simulink model "auto_pilot_upl"  (R2022b)
settings: Solver=FixedStepAuto  StartTime=0.0  StopTime=Inf  FixedStep=0.001  RelTol=1e-3  EnableMultiTasking=on
InitFcn:
  | clear mex
model workspace (MAT data in the model file):
  worldsim_instance : object (value not decoded)
values from neighbouring files (symbols this model uses):
  ACC_Adaptive_D = 0    [AutoPilot_parameters.m]    (also in ap_ini_param.mat; ap_initialModel.sldd = 0.0)
  ACC_Adaptive_I = 0    [AutoPilot_parameters.m]    (also in ap_ini_param.mat; ap_initialModel.sldd = 0.0)
  ACC_Adaptive_P = [5 7.5]    [AutoPilot_parameters.m]    (also in ap_ini_param.mat; ap_initialModel.sldd = 5.0 7.5)
  ACC_Classic_I = 5    [AutoPilot_parameters.m]    (also in ap_ini_param.mat; ap_initialModel.sldd = 5.0)
  ACC_Classic_P = 15    [AutoPilot_parameters.m]    (also in ap_ini_param.mat; ap_initialModel.sldd = 15.0)
  ACC_MaxBrake = 50    [AutoPilot_parameters.m]    (also in ap_ini_param.mat; ap_initialModel.sldd = 50.0)
  ACC_MaxThrottle = 130    [AutoPilot_parameters.m]    (also in ap_ini_param.mat = 80; ap_initialModel.sldd = 130.0)
  ACC_Module_Activity_Flag = 1    [AutoPilot_parameters.m]    (also in ap_ini_param.mat; ap_initialModel.sldd = 1.0)
  ACC_Ready_Speed = 30    [AutoPilot_parameters.m]    (also in ap_ini_param.mat; ap_initialModel.sldd = 30.0)
  ACC_SensorMaxDistance = 250    [AutoPilot_parameters.m]    (also in ap_ini_param.mat = 120; ap_initialModel.sldd = 250.0)
  ACC_Speed_Distance_control = 3    [AutoPilot_parameters.m]    (also in ap_ini_param.mat; ap_initialModel.sldd = 3.0)
  ACC_Speed_Distance_Gain = [0.1 0.15 0.2 0.25]    [AutoPilot_parameters.m]    (also in ap_ini_param.mat; ap_initialModel.sldd = 0.1 0.15 0.2 0.25)
  ADAS_Control_Mode = 1    [AutoPilot_parameters.m]    (also in ap_ini_param.mat; ap_initialModel.sldd = 1.0)
  AEB_Alarm_Freq = 5    [AutoPilot_parameters.m]    (also in ap_ini_param.mat; ap_initialModel.sldd = 5.0)
  AEB_Distance_To_Collision_Brake = 5    [AutoPilot_parameters.m]    (also in ap_ini_param.mat; ap_initialModel.sldd = 5.0)
  AEB_Freq_Hz = Sensor_Freq_worldsim/2    (= 25)    [AutoPilot_parameters.m]    (also in ap_ini_param.mat; ap_initialModel.sldd = 25.0)
  AEB_Gain = [1 1]    [AutoPilot_parameters.m]    (also in ap_ini_param.mat; ap_initialModel.sldd = 1.0 1.0)
  AEB_Gain_set = 60    [AutoPilot_parameters.m]    (also in ap_ini_param.mat; ap_initialModel.sldd = 60.0)
  AEB_Gain_set_mult = 0.03    [AutoPilot_parameters.m]    (also in ap_ini_param.mat; ap_initialModel.sldd)
  AEB_Max_Decel = [8 15]    [AutoPilot_parameters.m]    (also in ap_ini_param.mat; ap_initialModel.sldd = 8.0 15.0)
  AEB_Max_Speed = 150    [AutoPilot_parameters.m]    (also in ap_ini_param.mat = 100; ap_initialModel.sldd = 150.0)
  AEB_Min_Distance_at_Stop = 1    [AutoPilot_parameters.m]    (also in ap_ini_param.mat; ap_initialModel.sldd = 1.0)
  AEB_Module_Activity_Flag = 1    [AutoPilot_parameters.m]    (also in ap_ini_param.mat; ap_initialModel.sldd = 1.0)
  AEB_Pedestrian_type = 68    [AutoPilot_parameters.m]    (also in ap_ini_param.mat; ap_initialModel.sldd = 68.0)
  AEB_Steer_Max = 180    [AutoPilot_parameters.m]    (also in ap_ini_param.mat; ap_initialModel.sldd = 180.0)
  AP_Activity_Flag = 1    [AutoPilot_parameters.m]    (also in ap_ini_param.mat; ap_initialModel.sldd = 1.0)
  AP_D = [0.3 0.3]    [AutoPilot_parameters.m]    (also in ap_ini_param.mat; ap_initialModel.sldd = 0.3 0.3)
  AP_Dyn_Rate_Limiter_Gain = 0.1    [AutoPilot_parameters.m]    (also in ap_ini_param.mat; ap_initialModel.sldd)
  AP_Dyn_Rate_Limiter_Power = 10    [AutoPilot_parameters.m]    (also in ap_ini_param.mat; ap_initialModel.sldd = 10.0)
  AP_Error_Max = 3    [AutoPilot_parameters.m]    (also in ap_ini_param.mat; ap_initialModel.sldd = 3.0)
  AP_Freq_Hz = Sensor_Freq_worldsim    (= 50)    [AutoPilot_parameters.m]    (also in ap_ini_param.mat; ap_initialModel.sldd = 50.0)
  AP_I = [0.05 0.05]    [AutoPilot_parameters.m]    (also in ap_ini_param.mat; ap_initialModel.sldd = 0.05 0.05)
  AP_Max_Error_dydt_Disable = 0.5    [AutoPilot_parameters.m]    (also in ap_ini_param.mat; ap_initialModel.sldd)
  AP_On_Request_Time = 0.01    [AutoPilot_parameters.m]    (also in ap_ini_param.mat; ap_initialModel.sldd)
  AP_P = [0.2 0.2]    [AutoPilot_parameters.m]    (also in ap_ini_param.mat; ap_initialModel.sldd = 0.2 0.2)
  AP_Steer_Error_Max = 0.7    [AutoPilot_parameters.m]    (also in ap_ini_param.mat; ap_initialModel.sldd)
  AP_Steer_Rate_Max_radps = 1    [AutoPilot_parameters.m]    (also in ap_ini_param.mat; ap_initialModel.sldd = 1.0)
  AP_Transition_Rate = 0.5    [AutoPilot_parameters.m]    (also in ap_ini_param.mat; ap_initialModel.sldd)
  butter_a = [1 -1.9911142922 0.991153595869]    [ap_ini_param.mat]    (also in ap_initialModel.sldd = 1.0 -1.9911142922016536 0.99115359586893548)
  butter_b = [9.82591682048e-06 1.9651833641e-05 9.82591682048e-06]    [ap_ini_param.mat]    (also in ap_initialModel.sldd = 9.825916820482009E-6 1.9651833640964018E-5 9.825916820482009)
  Lane_Width = 3.7    [AutoPilot_parameters.m]    (also in ap_ini_param.mat; ap_initialModel.sldd)
  No_Target_Display_Value = 0    [AutoPilot_parameters.m]    (also in ap_ini_param.mat; ap_initialModel.sldd = 0.0)
  radar_source = 2    [AutoPilot_parameters.m]    (also in ap_ini_param.mat; ap_initialModel.sldd = 2.0)
  Sensor_Freq_worldsim = 50    [AutoPilot_parameters.m]    (also in ap_ini_param.mat; ap_initialModel.sldd = 50.0; launcher.m)
  stop_number_collisions = 10.0    [ap_initialModel.sldd]    (also in launcher.m = 10)
  stop_speed = 0.001    [ap_initialModel.sldd]    (also in launcher.m)
  stop_time = 12.0    [ap_initialModel.sldd]    (also in launcher.m = 12)
  vehicle_width = 2.2    [AutoPilot_parameters.m]    (also in ap_ini_param.mat = 1.86; ap_initialModel.sldd)
undefined symbols (not defined in the file or in its folder): light_brake_center, light_brake_left, light_brake_right
libraries: simulink x91, simwbSfunlib x49, viworldsim_lib x6, slpidlib x4
(part 4 of 4)

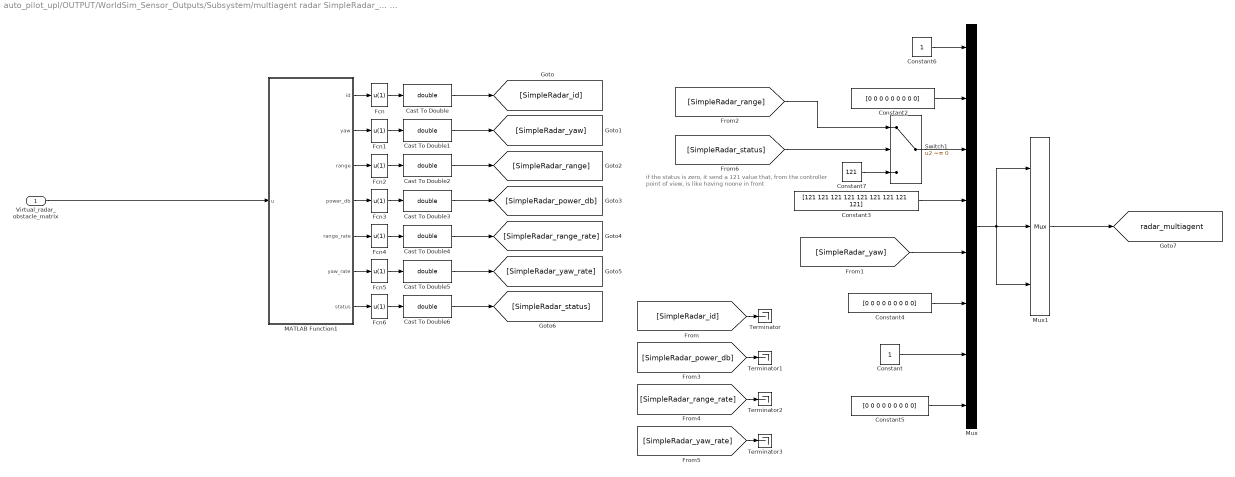
== system auto_pilot_upl/OUTPUT/WorldSim_Sensor_Outputs/Subsystem/multiagent radar SimpleRadar_... are single double representing id, yaw, range, power_db, range_rate, yaw_rate, status ==
  note: if the status is zero, it send a 121 value that,
      | from the controller point of view, is like having noone in front
  Virtual_radar_obstacle_matrix : Inport
  Cast To Double{,1..6} (7 alike) : DataTypeConversion  OutDataTypeStr=double  SaturateOnIntegerOverflow=off  RndMeth=Floor
  Constant : Constant
  Constant2 : Constant  Value=[0 0 0 0 0 0 0 0 0]
  Constant3 : Constant  Value=[121 121 121 121 121 121 121 121 121]
  Constant4 : Constant  Value=[0 0 0 0 0 0 0 0 0]
  Constant5 : Constant  Value=[0 0 0 0 0 0 0 0 0]
  Constant6 : Constant
  Constant7 : Constant  Value=121
  Fcn{,1..6} (7 alike) : Fcn  Expr=u(1)
  MATLAB Function1 : MATLAB Function  TreatAsAtomicUnit=on
  Mux : Mux  Inputs=8
  Mux1 : Mux  Inputs=3
  Switch1 : Switch  Criteria=u2 ~= 0  SaturateOnIntegerOverflow=off  InputSameDT=off
  Terminator{,1..3} (4 alike) : Terminator
  tag scope: radar_multiagent=global
  wires:
  Virtual_radar_obstacle_matrix/1 -> MATLAB Function1/1(u)
  MATLAB Function1/6(yaw_rate) -> Fcn5/1
  Cast To Double3/1 -> [SimpleRadar_power_db]
  Cast To Double5/1 -> [SimpleRadar_yaw_rate]
  MATLAB Function1/1(id) -> Fcn/1
  Fcn4/1 -> Cast To Double4/1
  Cast To Double2/1 -> [SimpleRadar_range]
  Fcn5/1 -> Cast To Double5/1
  MATLAB Function1/2(yaw) -> Fcn1/1
  Cast To Double/1 -> [SimpleRadar_id]
  MATLAB Function1/7(status) -> Fcn6/1
  Fcn1/1 -> Cast To Double1/1
  Fcn6/1 -> Cast To Double6/1
  Fcn/1 -> Cast To Double/1
  Cast To Double4/1 -> [SimpleRadar_range_rate]
  MATLAB Function1/5(range_rate) -> Fcn4/1
  Cast To Double1/1 -> [SimpleRadar_yaw]
  MATLAB Function1/4(power_db) -> Fcn3/1
  Fcn2/1 -> Cast To Double2/1
  Fcn3/1 -> Cast To Double3/1
  MATLAB Function1/3(range) -> Fcn2/1
  Cast To Double6/1 -> [SimpleRadar_status]
  Switch1/1 -> Mux/3
  [SimpleRadar_yaw] -> Mux/5
  [SimpleRadar_status] -> Switch1/2
  Constant3/1 -> Mux/4
  Mux/1 -> Mux1/3, Mux1/1, Mux1/2
  Constant5/1 -> Mux/8
  Constant6/1 -> Mux/1
  Constant/1 -> Mux/7
  Constant4/1 -> Mux/6
  [SimpleRadar_yaw_rate] -> Terminator3/1
  Constant7/1 -> Switch1/3
  Constant2/1 -> Mux/2
  [SimpleRadar_range_rate] -> Terminator2/1
  [SimpleRadar_range] -> Switch1/1
  Mux1/1 -> [radar_multiagent]
  [SimpleRadar_id] -> Terminator/1
  [SimpleRadar_power_db] -> Terminator1/1

== system auto_pilot_upl/OUTPUT/WorldSim_Sensor_Outputs/Subsystem/obstacle detection  ==
  Virtual_camera_obstacle_matrix : Inport
  From1 : From  Commented=on  GotoTag=Obstacles_id
  Gain : Gain  Gain=0.5
  MATLAB Function : MATLAB Function  TreatAsAtomicUnit=on
  MATLAB Function2 : MATLAB Function  TreatAsAtomicUnit=on
  Mux2 : Mux
  Mux3 : Mux  Inputs=3
  Sum : Sum  Inputs=+-
  Terminator{,4..8} (6 alike) : Terminator
  tag scope: Obstacles_nearest_point_x=global, Obstacles_nearest_point_y=global, Obstacles_nearest_point_z=global, Obstacles_type=global, radar_virtual=global
  wires:
  MATLAB Function2/1(tag) -> [Obstacles_type]
  Virtual_camera_obstacle_matrix/1 -> MATLAB Function2/1(u)
  Mux3/1 -> [radar_virtual]
  [Obstacles_nearest_point_x] -> MATLAB Function/1(x)
  [Obstacles_type] -> Mux2/4
  Mux2/1 -> Mux3/2, Mux3/1, Mux3/3
  [Obstacles_nearest_point_y] -> MATLAB Function/2(y)
  MATLAB Function/1(distanceToCollision) -> Mux2/2
  [Obstacles_type] -> Mux2/1
  [Obstacles_nearest_point_z] -> Terminator/1
  MATLAB Function/2(yaw) -> Mux2/3
  MATLAB Function2/3(center_y) -> [Obstacles_nearest_point_y]
  MATLAB Function2/4(center_z) -> [Obstacles_nearest_point_z]
  MATLAB Function2/5(center_rotation_x) -> Terminator6/1
  MATLAB Function2/6(center_rotation_y) -> Terminator7/1
  MATLAB Function2/7(center_rotation_z) -> Terminator8/1
  MATLAB Function2/9(size_y) -> Terminator4/1
  MATLAB Function2/10(size_z) -> Terminator5/1
  MATLAB Function2/8(size_x) -> Gain/1
  MATLAB Function2/2(center_x) -> Sum/1
  Gain/1 -> Sum/2
  Sum/1 -> [Obstacles_nearest_point_x]

== system auto_pilot_upl/OUTPUT/WorldSim_Sensor_Outputs/Subsystem/lane marking acquisition/derivation_speed ==
  Distance : Inport
  Trigger : TriggerPort  VariantControl=Variant  PortDimensions=1
  Discrete Derivative : simulink/Discrete/Discrete Derivative  gainval=1.0  ICPrevScaledInput=0.0  OutMin=[]  OutMax=[]  OutDataType=fixdt(1, 16)  OutScaling=2^-10  DoSatur=off
  Gain : Gain  Gain=-1
  Speed_of_approaching : Outport
  wires:
  Discrete Derivative/1 -> Gain/1
  Gain/1 -> Speed_of_approaching/1
  Distance/1 -> Discrete Derivative/1

== matlab function auto_pilot_upl/OUTPUT/WorldSim_Sensor_Outputs/Subsystem/obstacle detection /MATLAB Function2 ==
  data: u input; tag output; center_x output; center_y output; center_z output; center_rotation_x output; center_rotation_y output; center_rotation_z output; size_x output; size_y output; size_z output
function [tag, center_x, center_y, center_z, center_rotation_x, center_rotation_y, center_rotation_z, size_x, size_y, size_z] = fcn(u)

% this is the id tag that is assigned by ws at every scenario load
tag = (u(1,:))';
center_x = (u(2,:))';
center_y = (u(3,:))';
center_z = (u(4,:))';
center_rotation_x = (u(5,:))';
center_rotation_y = (u(6,:))';
center_rotation_z = (u(7,:))';
size_x = (u(8,:))';
size_y = (u(9,:))';
size_z = (u(10,:))';

%% identification of nearest box

% [index,index2]=min(u(:,3));
% 
% id = u(index,1);
% type = u(index,2);
% center_x = u(index,3);
% center_y = u(index,4);
% center_z = u(index,5);
% width = u(index,6);
% height = u(index,7);

== matlab function auto_pilot_upl/OUTPUT/WorldSim_Sensor_Outputs/Subsystem/obstacle detection /MATLAB Function ==
  data: x input; distanceToCollision output; y input; yaw output
function [distanceToCollision, yaw] = fcn(x, y)

x(x==0)=121;
y(y==0)=121;

yaw = atan(y./x);
distanceToCollision=x./cos(yaw);
distanceToCollision(x==121)=121;

== matlab function auto_pilot_upl/AEB/AEB_Inputs/MATLAB Function ==
  data: u input; y output
function y = fcn(u)

y = u;
y(u==121)=0;

== matlab function auto_pilot_upl/AEB/AEB_Inputs/MATLAB Function1 ==
  data: u input; y output
function y = fcn(u)

y = u;
y(u==121)=0;

== matlab function auto_pilot_upl/OUTPUT/WorldSim_Sensor_Outputs/Subsystem/bsd setection from ostacle recognition/MATLAB Function3 ==
  data: u input; semitrack input; left output; right output
function [left, right] = fcn(u, semitrack)
left=0;
right=0;

% [x,index] = min(nonzeros(u(:,3)));
x = (u(2,:))';
y = (u(3,:))';
% yaw = atan(y./x);
% distanceToCollision=x./cos(yaw);
index_left=find((y < -semitrack).*(y > -5),1);
index_right=find((y > semitrack).*(y < 5),1);
% .*(y > -3).*(x < 25)
if (~isempty(index_left))
    left = 1;
end
if (~isempty(index_right))
    right=1;
end

== matlab function auto_pilot_upl/OUTPUT/WorldSim_Sensor_Outputs/manipulation_of_objects1 ==
  data: complete_obstacles_matrix input; filtered_matrix output; detected_objects input
function filtered_matrix = fcn(complete_obstacles_matrix, detected_objects)

% computations

filtered_matrix = complete_obstacles_matrix;

filtered_matrix(:,((detected_objects+1):size(filtered_matrix,2))) = 0;

== matlab function auto_pilot_upl/AP/AP_Logic/MATLAB Function ==
  data: u input; y output
function y = fcn(u)

if u == 0
    y=1e-6;
else
    y=u;
end

end

== matlab function auto_pilot_upl/ACC/ACC_Logic/ACC_Target_Acquisition/SensorTargets_300000_InCurvedLane_mux/MATLAB Function ==
  data: Front_Axle_Steer input; Radius output; Rn output; wheelbase input; SensorTargets_300000_LongitudinalDistance input; SensorTargets_300000_LateralDistance input
function [Radius,Rn]= fcn(Front_Axle_Steer,wheelbase,SensorTargets_300000_LongitudinalDistance,SensorTargets_300000_LateralDistance)
%% Calc corner radius from steer at front axle
Radius = wheelbase./sin(Front_Axle_Steer) ; % (m)

%% Calc center of cirle coordinates (orgin reference at center of front axle)
yc = wheelbase./tan(Front_Axle_Steer) ; %(rad)
xc = -wheelbase ; %(m)

%% Calc target distance from circle center 
yn = SensorTargets_300000_LateralDistance ; %(m)
xn = SensorTargets_300000_LongitudinalDistance ; %(m)

Rn = sqrt((yn-yc).^2+(xn-xc).^2) ; %(m)

== matlab function auto_pilot_upl/OUTPUT/WorldSim_Sensor_Outputs/MATLAB Function ==
  data: lane_coefficiants input; left_lane_distance output; right_lane_distance output
function [left_lane_distance, right_lane_distance] = fcn(lane_coefficiants)

left_lane_distance = lane_coefficiants(1,1);
right_lane_distance = lane_coefficiants(2,1);

== matlab function auto_pilot_upl/OUTPUT/WorldSim_Sensor_Outputs/manipulation_of_objects ==
  data: complete_obstacles_matrix input; filtered_matrix output; detected_objects input
function filtered_matrix = fcn(complete_obstacles_matrix, detected_objects)

% computations

filtered_matrix = complete_obstacles_matrix;

filtered_matrix(:,((detected_objects+1):size(filtered_matrix,2))) = 0;

== matlab function auto_pilot_upl/ACC/ACC_Logic/ACC_Target_Acquisition/SensorTargets_300000_LateralDistance_mux/Target_Lateral_Position ==
  data: Target_distance input; Target_Lateral_Position output; Target_azimuth input
function Target_Lateral_Position = Target_Lateral_Position(Target_distance,Target_azimuth)
%#codegen

Target_Lateral_Position = Target_distance .* sin(Target_azimuth) ;

== matlab function auto_pilot_upl/ACC/ACC_Logic/ACC_Target_Acquisition/SensorTargets_300000_LongitudinalDistance_mux/Target_Longitudinal_Position ==
  data: Target_distance input; Target_Longitudinal_Position output; Target_azimuth input
function Target_Longitudinal_Position = Target_Longitudinal_Position(Target_distance,Target_azimuth)
%#codegen

Target_Longitudinal_Position = Target_distance .* cos(Target_azimuth) ;

== matlab function auto_pilot_upl/AEB/AEB_Logic/MATLAB Function ==
  data: distances_to_collision input; min_distance output
function min_distance = fcn(distances_to_collision)

temp = nonzeros(distances_to_collision);
if isempty(temp)
    min_distance = 121;
else
    min_distance = min(temp);
end

== matlab function auto_pilot_upl/AEB/AEB_Logic/Target_XY_Distance ==
  data: Target_distance_mux input; Target_Y_Distance_mux output; Target_azimuth_mux input; Target_X_Distance_mux output
function [Target_Y_Distance_mux,Target_X_Distance_mux] = Target_XY_Distance(Target_distance_mux,Target_azimuth_mux)
%#codegen

Target_Y_Distance_mux = Target_distance_mux .* sin(Target_azimuth_mux) ;
Target_X_Distance_mux = Target_distance_mux .* cos(Target_azimuth_mux) ;

== matlab function auto_pilot_upl/OUTPUT/WorldSim_Sensor_Outputs/Subsystem/multiagent radar SimpleRadar_... are single double representing id, yaw, range, power_db, range_rate, yaw_rate, status/MATLAB Function1 ==
  data: u input; id output; yaw output; range output; power_db output; range_rate output; yaw_rate output; status output
function [id, yaw, range, power_db, range_rate, yaw_rate,status] = fcn(u)

id = u(:,1);
yaw = u(:,2);
range = u(:,3);
power_db = u(:,4);
range_rate = u(:,5);
yaw_rate = u(:,6);
status = u(:,7);
